simulink model "IKS02A1_VL53L1A1_Both_ROS_fromworkspace_2025b_forstudents"  (R2025a)
settings: Solver=VariableStepAuto  StartTime=0.0  StopTime=sensorLog.GT_time.time(end)  RelTol=1e-3
settings Model: Creator=abich  LastModifiedBy=hsken

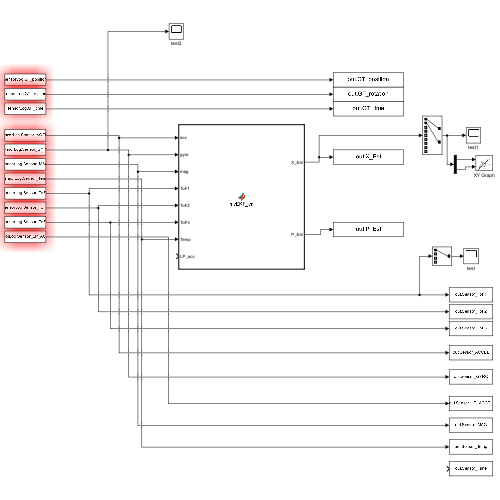
[thumbnail: Simulink's stored preview of the top-level diagram]
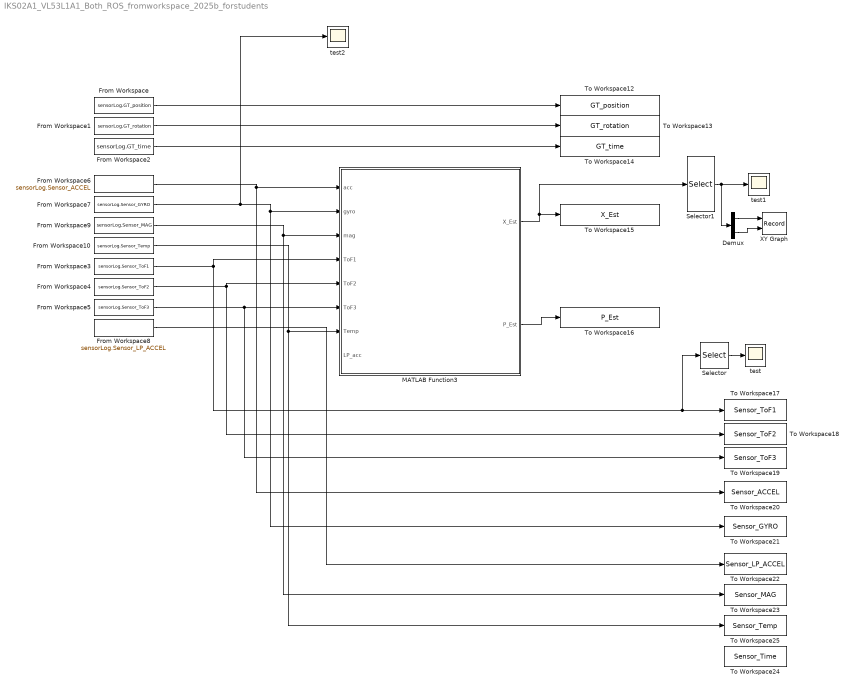
== system IKS02A1_VL53L1A1_Both_ROS_fromworkspace_2025b_forstudents ==
  Demux : Demux  Outputs=2
  From Workspace : FromWorkspace  VariableName=sensorLog.GT_position  SampleTime=1/200  OutputAfterFinalValue=Holding final value
  From Workspace1 : FromWorkspace  VariableName=sensorLog.GT_rotation  SampleTime=1/200  OutputAfterFinalValue=Holding final value
  From Workspace10 : FromWorkspace  VariableName=sensorLog.Sensor_Temp  SampleTime=1/200  OutputAfterFinalValue=Holding final value
  From Workspace2 : FromWorkspace  VariableName=sensorLog.GT_time  SampleTime=1/200  OutputAfterFinalValue=Holding final value
  From Workspace3 : FromWorkspace  VariableName=sensorLog.Sensor_ToF1  SampleTime=1/200  OutputAfterFinalValue=Holding final value
  From Workspace4 : FromWorkspace  VariableName=sensorLog.Sensor_ToF2  SampleTime=1/200  OutputAfterFinalValue=Holding final value
  From Workspace5 : FromWorkspace  VariableName=sensorLog.Sensor_ToF3  SampleTime=1/200  OutputAfterFinalValue=Holding final value
  From Workspace6 : FromWorkspace  VariableName=sensorLog.Sensor_ACCEL  SampleTime=1/200  OutputAfterFinalValue=Holding final value
  From Workspace7 : FromWorkspace  VariableName=sensorLog.Sensor_GYRO  SampleTime=1/200  OutputAfterFinalValue=Holding final value
  From Workspace8 : FromWorkspace  VariableName=sensorLog.Sensor_LP_ACCEL  SampleTime=1/200  OutputAfterFinalValue=Holding final value
  From Workspace9 : FromWorkspace  VariableName=sensorLog.Sensor_MAG  SampleTime=1/200  OutputAfterFinalValue=Holding final value
  MATLAB Function3 : MATLAB Function  TreatAsAtomicUnit=on
  Selector : Selector  InputPortWidth=4  IndexOptions=Index vector (dialog)  Indices=[1]  OutputSizes=1
  Selector1 : Selector  InputPortWidth=9  IndexOptions=Index vector (dialog)  Indices=[1 2]  OutputSizes=1
  To Workspace12 : ToWorkspace  VariableName=GT_position  SaveFormat=Structure With Time  SampleTime=1/200
  To Workspace13 : ToWorkspace  VariableName=GT_rotation  SaveFormat=Structure With Time  SampleTime=1/200
  To Workspace14 : ToWorkspace  VariableName=GT_time  SaveFormat=Structure With Time  SampleTime=1/200
  To Workspace15 : ToWorkspace  VariableName=X_Est  SaveFormat=Structure With Time  SampleTime=1/200
  To Workspace16 : ToWorkspace  VariableName=P_Est  SaveFormat=Structure With Time  SampleTime=1/200
  To Workspace17 : ToWorkspace  VariableName=Sensor_ToF1  SaveFormat=Structure With Time  SampleTime=1/200
  To Workspace18 : ToWorkspace  VariableName=Sensor_ToF2  SaveFormat=Structure With Time  SampleTime=1/200
  To Workspace19 : ToWorkspace  VariableName=Sensor_ToF3  SaveFormat=Structure With Time  SampleTime=1/200
  To Workspace20 : ToWorkspace  VariableName=Sensor_ACCEL  SaveFormat=Structure With Time  SampleTime=1/200
  To Workspace21 : ToWorkspace  VariableName=Sensor_GYRO  SaveFormat=Structure With Time  SampleTime=1/200
  To Workspace22 : ToWorkspace  VariableName=Sensor_LP_ACCEL  SaveFormat=Structure With Time  SampleTime=1/200
  To Workspace23 : ToWorkspace  VariableName=Sensor_MAG  SaveFormat=Structure With Time  SampleTime=1/200
  To Workspace24 : ToWorkspace  VariableName=Sensor_Time  SaveFormat=Structure With Time  SampleTime=1/200
  To Workspace25 : ToWorkspace  VariableName=Sensor_Temp  SaveFormat=Structure With Time  SampleTime=1/200
  XY Graph : Record  NumPorts=2.0  FileSettingsInternal="{\"entries\":[{\"content\":{\"excelSettings\":{\"content\":{},\"type\":\"Streamout.ExcelSettings\"},\"parquetSettings\":{\"content\":{},\"type\":\"Streamout.ParquetSettings\"}},\"type\":\"Streamout.FileSettingStorage\",\"uuid\":\"\"}],\"packageUris\":[\"http:\\/\\/schema.mathworks.com\\/mf0\\/streamout_blocks\\/R2020a\"],\"version\":\"1.0\"}"  FrameSettings=[0, 0]  Layout=[1 1]  SignalsInternal="{\"entries\":[{\"content\":{\"signals\":[{\"content\":{\"blockPath\":[],\"dimensions\":[1],\"domain\":\"\",\"lineColor\":\"#a2142f\",\"plots\":[ 1 ],\"port\":1,\"signalID\":1,\"signalName\":\"Demux:1\"},\"type\":\"RecordBlkView.Signal\",\"uuid\":\"\"},{\"content\":{\"blockPath\":[],\"dimensions\":[1],\"domain\":\"\",\"lineColor\":\"#139fff\",\"plots\":[ 1 ],\"port\":2,\"signalID\":2,\"signalName\":\"Demux:2\"},\"type\":\"RecordBlkView.Signal\",\"uuid\":\"\"}]},\"type\":\"RecordBlkView.InputSignals\",\"uuid\":\"\"}],\"packageUris\":[\"http:\\/\\/schema.mathworks.com\\/mf0\\/streamout_blocks\\/R2020a\"],\"version\":\"1.0\"}"  VisualizationBindings="{\"xyplotplugin\":{\"info\":[{\"series\":[{\"bindingParametersList\":[{\"parameter\":\"X-Axis\",\"signalID\":1,\"signalName\":\"Demux:1\"},{\"parameter\":\"Y-Axis\",\"signalID\":2,\"signalName\":\"Demux:2\"}],\"seriesID\":0}],\"subplotID\":1}]}}"  CompatibilityTag=XY
  test : Scope
      settings: ActiveDisplayYMinimum=-1  ActiveDisplayYMaximum=1
  test1 : Scope
      settings: ActiveDisplayYMinimum=-1  ActiveDisplayYMaximum=1
  test2 : Scope
      settings: ActiveDisplayYMinimum=-0.15108420974985681  ActiveDisplayYMaximum=0.16772460685752888  DataLoggingVariableName=ScopeData2
  wires:
  From Workspace4/1 -> To Workspace18/1, MATLAB Function3/5(ToF2)
  From Workspace6/1 -> To Workspace20/1, MATLAB Function3/1(acc)
  From Workspace9/1 -> To Workspace23/1, MATLAB Function3/3(mag)
  From Workspace10/1 -> To Workspace25/1, MATLAB Function3/7(Temp)
  From Workspace2/1 -> To Workspace14/1
  From Workspace5/1 -> To Workspace19/1, MATLAB Function3/6(ToF3)
  From Workspace/1 -> To Workspace12/1
  MATLAB Function3/1(X_Est) -> Selector1/1, To Workspace15/1
  From Workspace8/1 -> To Workspace22/1
  From Workspace3/1 -> Selector/1, To Workspace17/1, MATLAB Function3/4(ToF1)
  From Workspace1/1 -> To Workspace13/1
  From Workspace7/1 -> test2/1, To Workspace21/1, MATLAB Function3/2(gyro)
  MATLAB Function3/2(P_Est) -> To Workspace16/1
  Selector/1 -> test/1
  Selector1/1 -> Demux/1, test1/1
  Demux/1 -> XY Graph/1
  Demux/2 -> XY Graph/2

== matlab function IKS02A1_VL53L1A1_Both_ROS_fromworkspace_2025b_forstudents/MATLAB Function3 ==
  data: acc input; X_Est output; gyro input; mag input; ToF1 input; ToF2 input; ToF3 input; P_Est output; Temp input; LP_acc input
function [X_Est, P_Est] = myEKF_ca(acc, gyro, mag, ToF1, ToF2, ToF3, Temp, LP_acc) %#ok<INUSD>
%MYEKF_CA  Extended Kalman Filter for a mecanum-wheel robot (2-D + heading).
%          Constant-acceleration system model, persistent-variable interface.
%
% [X_Est, P_Est] = myEKF_ca(acc, gyro, mag, ToF1, ToF2, ToF3, Temp, LP_acc)
%
% Called once per sample from Simulink / a real-time loop.
% Rename file + function to myEKF when replacing the batch version.
%
% ---------- State vector (8 × 1) ----------
%   X = [x; y; theta; vx; vy; omega; ax; ay]
%   x, y    : position in arena frame  [m]   (origin at arena centre)
%   theta   : heading                  [rad]
%   vx, vy  : velocity, world frame    [m/s]
%   omega   : yaw rate                 [rad/s]
%   ax, ay  : acceleration, world frame[m/s^2]
%
% ---------- System model ----------
%   Constant-acceleration kinematics; state propagated with fixed dt.
%
% ---------- Sensor inputs ----------
%   acc   [3×1]  accelerometer  – indices 2,3 are robot x,y body axes
%   gyro  [3×1]  gyroscope      – index  1   is yaw rate (vertical axis)
%   mag   [3×1]  magnetometer   – indices 2,3 give heading in xy plane
%   ToF1  [4×1]  left-facing    : ch1 = range [mm], ch4 = status (0 = ok)
%   ToF2  [4×1]  forward-facing : ch1 = range [mm], ch4 = status (0 = ok)
%   ToF3  [4×1]  right-facing   : ch1 = range [mm], ch4 = status (0 = ok)
%   Temp, LP_acc  – ignored
%
% ---------- Arena convention ----------
%   Rectangular arena centred at origin; walls at x = ±Lx, y = ±Ly.
%
% ---------- Board orientation ----------
%   Board is upended so that the robot's horizontal plane maps to sensor
%   indices 2 & 3:
%     acc(2), acc(3)  → body-frame x, y acceleration
%     gyro(1)         → yaw rate (rotation about the vertical axis)
%     mag(2), mag(3)  → heading components

% =========================================================================
%  PERSISTENT STATE
% =========================================================================
persistent X P Q R_imu R_tof initialised
persistent Lx Ly tof_offsets tof_phi
persistent acc_scale gyro_scale mag_declination dt
persistent chi2_thresh
persistent step mag_update_freq tof_update_freq
persistent acc_x_bias acc_y_bias gyro_x_bias gyro_y_bias mag_x_bias mag_y_bias

% =========================================================================
%  ONE-TIME INITIALISATION  ← edit all tuning / geometry here
% =========================================================================
if isempty(initialised)

    % --- Sample period [s] and sensor decimation ratios ------------------
    dt              = 1/200;   % EKF rate  [Hz]
    mag_update_freq = 4;       % mag  runs at 200/4  = 50 Hz
    tof_update_freq = 20;      % ToF  runs at 200/20 = 10 Hz
    step            = 0;

    % --- Arena full-dimensions [m]  (walls at x = ±Lx, y = ±Ly) ---------
    Lx = 2.44;
    Ly = 2.44;

    % --- Raw-sensor scaling ----------------------------------------------
    acc_scale       = 1.0;    % multiply raw acc  to get [m/s^2]
    gyro_scale      = 1.0;    % multiply raw gyro to get [rad/s]
    mag_declination = 1.248;  % add to atan2(mag) to align with world frame [rad]

    % --- ToF sensor offsets from robot centre, body frame [m] ------------
    %   Row i = [dx_fwd, dy_left]
    %     dx_fwd  > 0  →  toward robot front
    %     dy_left > 0  →  toward robot left side
    tof_offsets = [ 0.20,  0.04;   % ToF1 – right-facing
                    0.209, 0.00;   % ToF2 – forward-facing
                    0.20, -0.04];  % ToF3 – left-facing

    % --- ToF firing angles relative to body forward axis [rad] -----------
    tof_phi = [-pi/2; 0; pi/2];   % right, forward, left

    % --- Mahalanobis gate  (chi-sq 1 DOF, 99th percentile) --------------
    chi2_thresh = 6.63;

    % --- Initial state ---------------------------------------------------
    X = zeros(8, 1);   % assume robot starts at arena centre, at rest

    % --- Initial covariance P --------------------------------------------
    P = diag([ 0.50,  0.50,  deg2rad(45), ...   % x, y, theta
               0.50,  0.50,  0.20,        ...   % vx, vy, omega
               1.00,  1.00 ].^2);               % ax, ay

    % --- Process noise Q -------------------------------------------------
    Q = diag([ 5e-3, 5e-3, deg2rad(3), ...   % x, y, theta
               0.05, 0.05, 0.10,       ...   % vx, vy, omega
               0.30, 0.30 ].^2);             % ax, ay

    % --- IMU measurement noise  z = [acc_bx, acc_by, omega, heading] ----
    % Gyro/acc trusted tightly; mag noise large so it only prevents drift
    R_imu = diag([ 0.50, 0.50, 0.02, deg2rad(45) ].^2);

    % --- ToF measurement noise [m^2] -------------------------------------
    R_tof = (0.05)^2;

    % --- Sensor Calibrations ---------------------------------------------
    acc_x_bias = 0.0275;      acc_y_bias = -0.3963;
    gyro_x_bias = -0.0112;    gyro_y_bias = -0.0013;
    mag_x_bias = -5.4548e-05; mag_y_bias = 8.6087e-05;

    initialised = true;
end

% =========================================================================
%  STEP COUNTER  (drives sensor decimation)
% =========================================================================
step = step + 1;

do_mag = (mod(step, mag_update_freq) == 0);   % true every 4th  call (50 Hz)
do_tof = (mod(step, tof_update_freq) == 0);   % true every 20th call (10 Hz)

% =========================================================================
%  EXTRACT MEASUREMENTS
% =========================================================================
% Board upended: robot horizontal plane on sensor indices 2 & 3
acc_bx = double(acc(2))  * acc_scale - acc_x_bias;    % body x-acceleration  [m/s^2]
acc_by = double(acc(3))  * acc_scale - acc_y_bias;    % body y-acceleration  [m/s^2]
gyro_z = double(gyro(1)) * gyro_scale - gyro_x_bias;  % yaw rate             [rad/s]

% Magnetometer heading (horizontal components on indices 2 & 3)
mag_heading = -atan2(double(mag(3) - mag_y_bias), double(mag(2) - mag_x_bias)) + mag_declination;

% ToF: channel 1 = range (m), channel 4 = status (0 = valid)
tof_d  = double([ToF1(1); ToF2(1); ToF3(1)]);
tof_ok = double([ToF1(4); ToF2(4); ToF3(4)]) == 0;

% =========================================================================
%  PREDICTION STEP  — constant acceleration
% =========================================================================
x_s = X(1);  y_s = X(2);  th  = X(3);
vx  = X(4);  vy  = X(5);  om  = X(6);
axw = X(7);  ayw = X(8);

X_p = [
    x_s + vx*dt + 0.5*axw*dt^2;
    y_s + vy*dt + 0.5*ayw*dt^2;
    wrapToPi(th + om*dt);
    vx  + axw*dt;
    vy  + ayw*dt;
    om;
    axw;
    ayw
];

% State-transition Jacobian  F = ∂f/∂X
F      = eye(8);
F(1,4) = dt;    F(1,7) = 0.5*dt^2;
F(2,5) = dt;    F(2,8) = 0.5*dt^2;
F(3,6) = dt;
F(4,7) = dt;
F(5,8) = dt;

P_p = F * P * F' + Q;

% =========================================================================
%  UPDATE — IMU  (acc + gyro every step;  magnetometer at 50 Hz)
% =========================================================================
th_p = X_p(3);
axp  = X_p(7);
ayp  = X_p(8);
omp  = X_p(6);

% Predicted body-frame accelerations  (world → body rotation)
h_ax  =  axp*cos(th_p) + ayp*sin(th_p);
h_ay  = -axp*sin(th_p) + ayp*cos(th_p);

if do_mag
    % Full update: acc_bx, acc_by, gyro_z, mag_heading  [4 measurements]
    h_imu = [h_ax; h_ay; omp; th_p];

    H_imu = zeros(4, 8);
    H_imu(1,3) = -axp*sin(th_p) + ayp*cos(th_p);    % ∂h_ax/∂theta
    H_imu(1,7) =  cos(th_p);                        % ∂h_ax/∂ax
    H_imu(1,8) =  sin(th_p);                        % ∂h_ax/∂ay
    H_imu(2,3) = -axp*cos(th_p) - ayp*sin(th_p);    % ∂h_ay/∂theta
    H_imu(2,7) = -sin(th_p);                        % ∂h_ay/∂ax
    H_imu(2,8) =  cos(th_p);                        % ∂h_ay/∂ay
    H_imu(3,6) =  1;                                % ∂omega/∂omega
    H_imu(4,3) =  1;                                % ∂theta/∂theta

    z_imu     = [acc_bx; acc_by; gyro_z; mag_heading];
    nu_imu    = z_imu - h_imu;
    nu_imu(4) = wrapToPi(nu_imu(4));

    R_upd = R_imu;

    S_imu = H_imu * P_p * H_imu' + R_upd;
    K_imu = P_p * H_imu' / S_imu;

    X_u    = X_p + K_imu * nu_imu;
    X_u(3) = wrapToPi(X_u(3));
    P_u    = (eye(8) - K_imu * H_imu) * P_p;
else
    % Partial update: acc_bx, acc_by, gyro_z only  [3 measurements]
    h_imu = [h_ax; h_ay; omp];

    H_imu = zeros(3, 8);
    H_imu(1,3) = -axp*sin(th_p) + ayp*cos(th_p);
    H_imu(1,7) =  cos(th_p);
    H_imu(1,8) =  sin(th_p);
    H_imu(2,3) = -axp*cos(th_p) - ayp*sin(th_p);
    H_imu(2,7) = -sin(th_p);
    H_imu(2,8) =  cos(th_p);
    H_imu(3,6) =  1;

    z_imu  = [acc_bx; acc_by; gyro_z];
    nu_imu = z_imu - h_imu;

    R_upd = R_imu(1:3, 1:3);

    S_imu = H_imu * P_p * H_imu' + R_upd;
    K_imu = P_p * H_imu' / S_imu;

    X_u    = X_p + K_imu * nu_imu;
    X_u(3) = wrapToPi(X_u(3));
    P_u    = (eye(8) - K_imu * H_imu) * P_p;
end
% 
% S_imu = H_imu * P_p * H_imu' + R_upd;
% K_imu = P_p * H_imu' / S_imu;
% 
% X_u    = X_p + K_imu * nu_imu;
% X_u(3) = wrapToPi(X_u(3));
% P_u    = (eye(8) - K_imu * H_imu) * P_p;

% =========================================================================
%  UPDATE — ToF sensors  (10 Hz: every 20th step)
% =========================================================================
for s = 1:3 * do_tof
    if ~tof_ok(s)
        continue
    end

    th_u    = X_u(3);
    dx_body = tof_offsets(s, 1);
    dy_body = tof_offsets(s, 2);

    % Sensor position in world frame
    sx = X_u(1) + cos(th_u)*dx_body - sin(th_u)*dy_body;
    sy = X_u(2) + sin(th_u)*dx_body + cos(th_u)*dy_body;

    % Predicted range and analytical Jacobian w.r.t. sensor pos & angle
    [h_pred, dh_dsx, dh_dsy, dh_dth_s] = tof_measurement( ...
        sx, sy, th_u, tof_phi(s), Lx, Ly);

    if h_pred <= 0
        continue
    end

    % ∂(sensor world pos)/∂theta via offset rotation
    dsx_dth = -sin(th_u)*dx_body - cos(th_u)*dy_body;
    dsy_dth =  cos(th_u)*dx_body - sin(th_u)*dy_body;

    % Full measurement Jacobian row  H_tof [1 × 8]
    H_tof    = zeros(1, 8);
    H_tof(1) = dh_dsx;                                         % ∂h/∂x
    H_tof(2) = dh_dsy;                                         % ∂h/∂y
    H_tof(3) = 0;   % ToF does not correct theta — heading left to gyro/mag

    nu_tof = tof_d(s) - h_pred;
    S_tof  = H_tof * P_u * H_tof' + R_tof;

    % Mahalanobis gate — rejects outliers (holes in walls, reflections, etc.)
    if (nu_tof^2 / S_tof) > chi2_thresh
        continue
    end

    K_tof  = P_u * H_tof' / S_tof;
    X_u    = X_u + K_tof * nu_tof;
    X_u(3) = wrapToPi(X_u(3));
    P_u    = (eye(8) - K_tof * H_tof) * P_u;
end

% =========================================================================
%  STORE STATE AND RETURN
% =========================================================================
X = X_u;
P = P_u;

X_Est = X;
P_Est = P;

end % myEKF_ca

% =========================================================================
%  LOCAL HELPER — analytical ToF range measurement model
% =========================================================================
function [h, dh_dsx, dh_dsy, dh_dth_s] = tof_measurement(sx, sy, th, phi_s, Lx, Ly)
%TOF_MEASUREMENT  Range from sensor world position (sx,sy) to nearest wall.
%
%   Arena walls at x = ±Lx, y = ±Ly (origin at centre).
%   Ray fired at world angle (th + phi_s).
%   Returns h (predicted range) and partial derivatives for EKF Jacobian.

    ray = th + phi_s;
    cd  = cos(ray);
    sd  = sin(ray);

    t = inf(4, 1);
    if abs(cd) > 1e-9
        t(1) = ( Lx - sx) / cd;   % wall x = +Lx
        t(2) = (-Lx - sx) / cd;   % wall x = -Lx
    end
    if abs(sd) > 1e-9
        t(3) = ( Ly - sy) / sd;   % wall y = +Ly
        t(4) = (-Ly - sy) / sd;   % wall y = -Ly
    end

    t(t <= 1e-6) = inf;            % discard behind-sensor intersections
    [h, wall] = min(t);

    if isinf(h)
        h = -1;  dh_dsx = 0;  dh_dsy = 0;  dh_dth_s = 0;
        return
    end

    % Analytical partial derivatives (depend on which wall was hit)
    switch wall
        case 1  % x = +Lx
            dh_dsx   = -1 / cd;
            dh_dsy   =  0;
            dh_dth_s =  ( Lx - sx) * sd / cd^2;
        case 2  % x = -Lx
            dh_dsx   = -1 / cd;
            dh_dsy   =  0;
            dh_dth_s =  (-Lx - sx) * sd / cd^2;
        case 3  % y = +Ly
            dh_dsx   =  0;
            dh_dsy   = -1 / sd;
            dh_dth_s = -( Ly - sy) * cd / sd^2;
        case 4  % y = -Ly
            dh_dsx   =  0;
            dh_dsy   = -1 / sd;
            dh_dth_s = -(-Ly - sy) * cd / sd^2;
        otherwise
            h = -1;  dh_dsx = 0;  dh_dsy = 0;  dh_dth_s = 0;
    end
end
